simulink model "kaffeeautomat_3"  (R2015b)
settings: Solver=FixedStepAuto  StartTime=0.0  StopTime=60  RelTol=1e-3
libraries: simulink x1
settings Model: Creator=scco1019  LastModifiedBy=scco1019

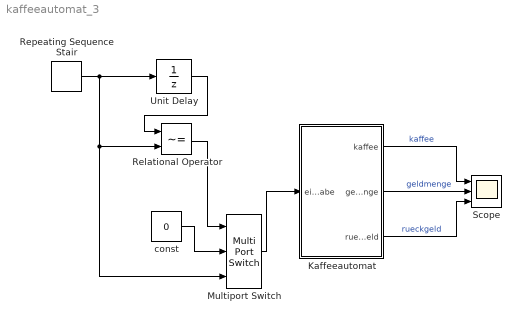
== system kaffeeautomat_3 ==
  Kaffeeautomat : Stateflow chart  TreatAsAtomicUnit=on
  Multiport Switch : MultiPortSwitch  DataPortOrder=Zero-based contiguous  Inputs=2
  Relational Operator : RelationalOperator  Operator=~=  OutDataTypeStr=boolean
  Repeating Sequence Stair : simulink/Sources/Repeating Sequence Stair  OutValues=[10 0 10 0 10 0 10 0 10 0 20 0 20 0 10 0 10 10 10 0 20 50 10 20 20 10 50].'  tsamp=-1  OutMin=[]  OutMax=[]  OutDataTypeStr=double  OutputDataTypeScalingMode=double  OutDataType=fixdt(0,8)  ConRadixGroup=Best Precision: Vector-wise  OutScaling=2^-12
  Scope : Scope  NumInputPorts=3
  Unit Delay : UnitDelay  SampleTime=-1
  "const " : Constant  Value=0
  wires:
  Multiport Switch/1 -> Kaffeeautomat/1(eingabe)
  Repeating Sequence Stair/1 -> Multiport Switch/3, Relational Operator/2, Unit Delay/1
  "const "/1 -> Multiport Switch/2
  Kaffeeautomat/2(geldmenge) -> Scope/2  "geldmenge"
  Kaffeeautomat/1(kaffee) -> Scope/1  "kaffee"
  Kaffeeautomat/3(rueckgeld) -> Scope/3  "rueckgeld"
  Unit Delay/1 -> Relational Operator/1
  Relational Operator/1 -> Multiport Switch/1

== stateflow chart kaffeeautomat_3/Kaffeeautomat ==
  state Kein_Kaffee/
    entry: kaffee=0;
    rueckgeld=0;
    geldmenge=geldmenge+eingabe;
  state Kaffee/
    entry: kaffee=1;
    entry: rueckgeld=geldmenge-50;
  (default) -> Kein_Kaffee : {geldmenge=0}
  Kein_Kaffee -> Kein_Kaffee [order 2]
  Kaffee -> Kein_Kaffee : {kaffee=0;
      | geldmenge=0;}
  Kein_Kaffee -> Kaffee [order 1] : [geldmenge>=50]
  data: eingabe input; kaffee output; geldmenge output; rueckgeld output
